simulink model "p3_w1_car"  (R2023b)
settings: Solver=FixedStepAuto  StartTime=0.0  StopTime=1370  FixedStep=0.01  RelTol=1e-3
values from neighbouring files (symbols this model uses):
  DriveData = [0 ... (first row only)    [initDriveCycle.m]
  Time = (0:1:1370)'    [initDriveCycle.m]
undefined symbols (not defined in the file or in its folder): C0, C1, C2, Iw, M, mph2mps, r
libraries: slpidlib x1
settings Model: Creator=anshu16  LastModifiedBy=lpoir
settings SolverCC: AlgebraicLoopSolver=TrustRegion
settings OptimizationCC: ReuseModelBlockBuffer=off
settings DebuggingCC: UnconnectedInputMsg=warning  UnconnectedOutputMsg=warning  UnconnectedLineMsg=warning
settings ModelReferenceCC: EnableRefExpFcnMdlSchedulingChecks=on
settings SFSimCC: CustomCodeUndefinedFunction=UseInterfaceOnly

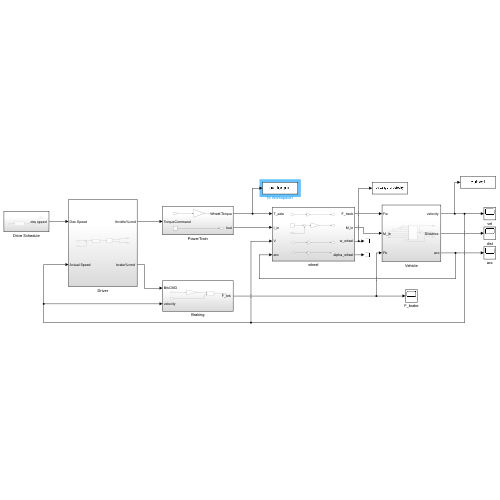
[thumbnail: Simulink's stored preview of the top-level diagram]
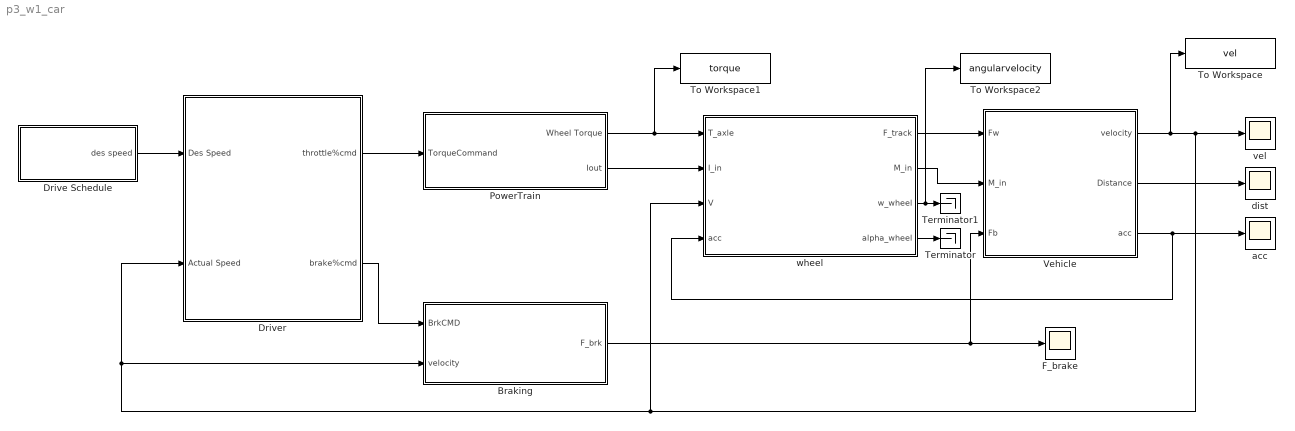
== system p3_w1_car ==
  Braking : Subsystem
  Drive Schedule : Subsystem
  "Driver " : Subsystem
  F_brake : Scope
  PowerTrain : Subsystem
  Terminator : Terminator
  Terminator1 : Terminator
  To Workspace : ToWorkspace  VariableName=vel  SaveFormat=Timeseries  SampleTime=-1
  To Workspace1 : ToWorkspace  VariableName=torque  SaveFormat=Timeseries  SampleTime=-1
  To Workspace2 : ToWorkspace  VariableName=angularvelocity  SaveFormat=Timeseries  SampleTime=-1
  Vehicle : Subsystem
  acc : Scope
  dist : Scope
  vel : Scope
  "wheel " : Subsystem
  wires:
  Drive Schedule/1("des speed ") -> "Driver "/1("Des Speed ")
  "Driver "/2("brake%cmd ") -> Braking/1("BrkCMD ")
  Braking/1("F_brk ") -> Vehicle/3("Fb "), F_brake/1
  Vehicle/3(acc) -> acc/1, "wheel "/4(acc)
  PowerTrain/1(Wheel Torque) -> To Workspace1/1, "wheel "/1(T_axle)
  PowerTrain/2(Iout) -> "wheel "/2(I_in)
  "wheel "/2(M_in) -> Vehicle/2("M_in ")
  "wheel "/1(F_track) -> Vehicle/1("Fw ")
  Vehicle/2("Distance ") -> dist/1
  Vehicle/1("velocity ") -> To Workspace/1, vel/1, "wheel "/3(V), "Driver "/2(Actual Speed), Braking/2("velocity ")
  "Driver "/1(throttle%cmd) -> PowerTrain/1(TorqueCommand)
  "wheel "/4(alpha_wheel) -> Terminator/1
  "wheel "/3(w_wheel) -> To Workspace2/1, Terminator1/1

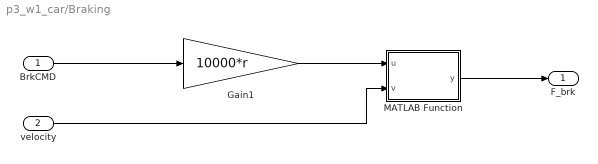
== system p3_w1_car/Braking ==
  "BrkCMD " : Inport
  "velocity " : Inport  Port=2
  Gain1 : Gain  Gain=10000*r
  MATLAB Function : MATLAB Function  TreatAsAtomicUnit=on
  "F_brk " : Outport  VectorParamsAs1DForOutWhenUnconnected=off
  wires:
  "BrkCMD "/1 -> Gain1/1
  Gain1/1 -> MATLAB Function/1(u)
  MATLAB Function/1(y) -> "F_brk "/1
  "velocity "/1 -> MATLAB Function/2(v)

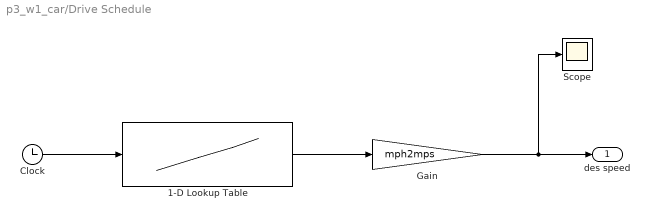
== system p3_w1_car/Drive Schedule ==
  1-D Lookup Table : Lookup_n-D  NumberOfTableDimensions=1  BreakpointsForDimension1=Time  Table=DriveData  InternalRulePriority=Speed  RndMeth=Simplest
  Clock : Clock
  Gain : Gain  Gain=mph2mps
  Scope : Scope
  "des speed " : Outport  VectorParamsAs1DForOutWhenUnconnected=off
  wires:
  Clock/1 -> 1-D Lookup Table/1
  1-D Lookup Table/1 -> Gain/1
  Gain/1 -> "des speed "/1, Scope/1

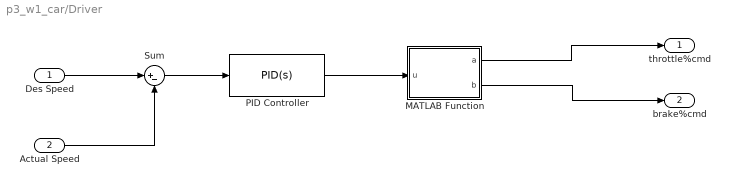
== system p3_w1_car/Driver  ==
  "Des Speed " : Inport
  Actual Speed : Inport  Port=2
  MATLAB Function : MATLAB Function  TreatAsAtomicUnit=on
  PID Controller : slpidlib/PID Controller  Controller=PID  Form=Parallel  TimeDomain=Continuous-time  UseExternalTs=off  SampleTime=-1  IntegratorMethod=Forward Euler  FilterMethod=Forward Euler  ControllerParametersSource=internal  P=0.5  I=0  UseKiTs=off  D=0  N=100  UseFilter=on  TunerSelectOption=Transfer Function Based (PID Tuner App)  InitialConditionSource=internal  InitialConditionForIntegrator=0  InitialConditionForFilter=0  DifferentiatorICPrevScaledInput=0  ExternalReset=none  TrackingMode=off  Kt=1  LimitOutput=on  SatLimitsSource=internal  UpperSaturationLimit=1  LowerSaturationLimit=-1  LinearizeAsGain=off  AntiWindupMode=none  Kb=1  LimitIntegrator=off  UpperIntegratorSaturationLimit=inf  LowerIntegratorSaturationLimit=-inf  POutMin=[]  POutMax=[]  IOutMin=[]  IOutMax=[]  DOutMin=[]  DOutMax=[]  NOutMin=[]  NOutMax=[]  SumOutMin=[]  SumOutMax=[]  SaturationOutMin=[]  SaturationOutMax=[]  PParamMin=[]  PParamMax=[]  IParamMin=[]  IParamMax=[]  DParamMin=[]  DParamMax=[]  NParamMin=[]  NParamMax=[]  KbParamMin=[]  KbParamMax=[]  KtParamMin=[]  KtParamMax=[]  KbOutMin=[]  KbOutMax=[]  KtOutMin=[]  KtOutMax=[]  IntegratorOutMin=[]  IntegratorOutMax=[]  FilterOutMin=[]  FilterOutMax=[]  SumI1OutMin=[]  SumI1OutMax=[]  SumI2OutMin=[]  SumI2OutMax=[]  SumI3OutMin=[]  SumI3OutMax=[]  SumI4OutMin=[]  SumI4OutMax=[]  SumDOutMin=[]  SumDOutMax=[]  DifferentiatorOutMin=[]  DifferentiatorOutMax=[]  FilterDiffOutCoefMin=[]  FilterDiffOutCoefMax=[]  ReciprocalOutMin=[]  ReciprocalOutMax=[]  SumDenOutMin=[]  SumDenOutMax=[]  SumNumOutMin=[]  SumNumOutMax=[]  DivideOutMin=[]  DivideOutMax=[]  UdiffTsProdOutMin=[]  UdiffTsProdOutMax=[]  NTsProdOutMin=[]  NTsProdOutMax=[]  UintegralTsProdOutMin=[]  UintegralTsProdOutMax=[]  UngainTsProdOutMin=[]  UngainTsProdOutMax=[]  ClampingZeroOutDataTypeStr=Inherit: Inherit via back propagation  ClampingZeroOutMin=[]  ClampingZeroOutMax=[]  FilterDenConstantOutDataTypeStr=Inherit: Inherit via back propagation  FilterDenConstantOutMin=[]  FilterDenConstantOutMax=[]  PCopyOutDataTypeStr=Inherit: Inherit via back propagation  PCopyOutMin=[]  PCopyOutMax=[]  NCopyOutDataTypeStr=Inherit: Inherit via back propagation  NCopyOutMin=[]  NCopyOutMax=[]  IntegratorContinuousStateAttributes=''  IntegratorStateMustResolveToSignalObject=off  IntegratorRTWStateStorageClass=Auto  FilterContinuousStateAttributes=''  FilterStateMustResolveToSignalObject=off  FilterRTWStateStorageClass=Auto  ParallelPVariant=InternalParameters  IdealPVariant=Disabled  IVariant=InternalParameters  DVariant=InternalParameters  IntegratorVariant=Continuous  SatVariant=Enabled  AWVariant=Passthrough  PCopyVariant=Disabled  TRVariant=Disabled  FdbkBlocksVariant=Forward  IdealPFdbkVariant=Disabled  SatFdbkVariant=Disabled  DerivativeFilterVariant=ContFilter  NVariant=InternalParameters  NCopyVariant=Disabled  FilterICVariant=InternalICsFilter  IntegratorICVariant=InternalICs  ExternalResetVariant=Disabled  TRSumVariant=Passthrough  SumFdbkVariant=Disabled  SumVariant=Sum_PID  TsampFilterVariant=InternalTs  TsampNgainVariant=Passthrough  TsampIntegralVariant=Disabled_SignalSpec  ExternalSaturationOutDataTypeStr=Inherit: Same as second input
  Sum : Sum  Inputs=|+-
  throttle%cmd : Outport
  "brake%cmd " : Outport  Port=2
  wires:
  "Des Speed "/1 -> Sum/1
  Actual Speed/1 -> Sum/2
  MATLAB Function/2(b) -> "brake%cmd "/1
  MATLAB Function/1(a) -> throttle%cmd/1
  Sum/1 -> PID Controller/1
  PID Controller/1 -> MATLAB Function/1(u)

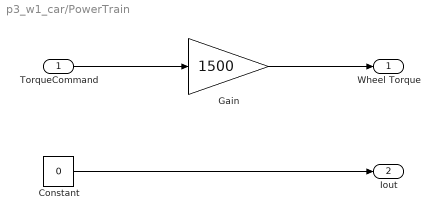
== system p3_w1_car/PowerTrain ==
  TorqueCommand : Inport
  Constant : Constant  Value=0
  Gain : Gain  Gain=1500
  Wheel Torque : Outport
  Iout : Outport  Port=2
  wires:
  TorqueCommand/1 -> Gain/1
  Gain/1 -> Wheel Torque/1
  Constant/1 -> Iout/1

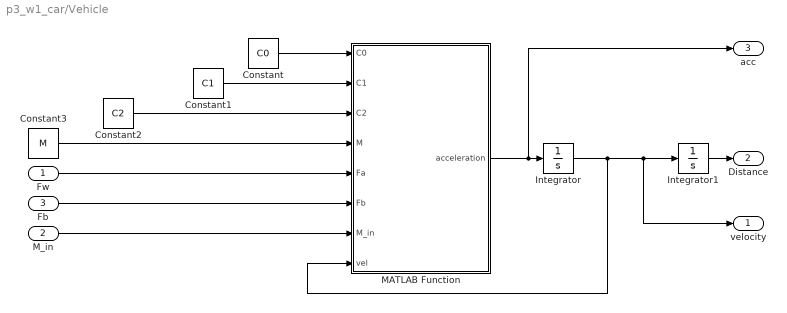
== system p3_w1_car/Vehicle ==
  "Fw " : Inport
  "M_in " : Inport  Port=2
  "Fb " : Inport  Port=3
  Constant : Constant  Value=C0
  Constant1 : Constant  Value=C1
  Constant2 : Constant  Value=C2
  Constant3 : Constant  Value=M
  Integrator : Integrator  LimitOutput=on  LowerSaturationLimit=0
  Integrator1 : Integrator
  MATLAB Function : MATLAB Function  TreatAsAtomicUnit=on
  "velocity " : Outport  VectorParamsAs1DForOutWhenUnconnected=off
  "Distance " : Outport  Port=2  VectorParamsAs1DForOutWhenUnconnected=off
  acc : Outport  Port=3
  wires:
  Constant1/1 -> MATLAB Function/2(C1)
  Constant/1 -> MATLAB Function/1(C0)
  MATLAB Function/1(acceleration) -> acc/1, Integrator/1
  Constant2/1 -> MATLAB Function/3(C2)
  Constant3/1 -> MATLAB Function/4(M)
  "Fw "/1 -> MATLAB Function/5(Fa)
  "Fb "/1 -> MATLAB Function/6(Fb)
  Integrator/1 -> MATLAB Function/8(vel), "velocity "/1, Integrator1/1
  Integrator1/1 -> "Distance "/1
  "M_in "/1 -> MATLAB Function/7(M_in)

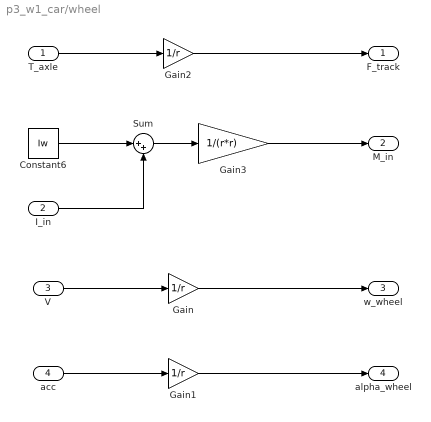
== system p3_w1_car/wheel  ==
  T_axle : Inport
  I_in : Inport  Port=2
  V : Inport  Port=3
  acc : Inport  Port=4
  Constant6 : Constant  Value=Iw
  Gain : Gain  Gain=1/r
  Gain1 : Gain  Gain=1/r
  Gain2 : Gain  Gain=1/r
  Gain3 : Gain  Gain=1/(r*r)
  Sum : Sum  Inputs=|++
  F_track : Outport
  M_in : Outport  Port=2
  w_wheel : Outport  Port=3
  alpha_wheel : Outport  Port=4
  wires:
  Gain/1 -> w_wheel/1
  V/1 -> Gain/1
  acc/1 -> Gain1/1
  Gain1/1 -> alpha_wheel/1
  T_axle/1 -> Gain2/1
  Gain2/1 -> F_track/1
  Gain3/1 -> M_in/1
  Constant6/1 -> Sum/1
  I_in/1 -> Sum/2
  Sum/1 -> Gain3/1

== matlab function p3_w1_car/Driver /MATLAB Function ==
  data: u input; a output; b output
function [a,b] = fcn(u)

if u>0
    acc=u;
    brk=0;
elseif u<0
    acc=0;
    brk=-u;
else
    acc=0;
    brk=0;
end
a= acc;
b= brk;

== matlab function p3_w1_car/Vehicle/MATLAB Function ==
  data: C0 input; acceleration output; C1 input; C2 input; M input; Fa input; Fb input; M_in input; vel input
function acceleration   = vehicle(C0,C1,C2,M,Fa,Fb,M_in, vel)

acceleration = (((Fa-Fb))-(C0+ C1*vel + C2*(vel)^2))/(M+M_in);

== matlab function p3_w1_car/Braking/MATLAB Function ==
  data: u input; y output; v input
function y = fcn(u,v)
%y =u*sign(v)
y = u * v/(abs(v)+0.001);
y = u;
